simulink model "mcb_open_loop_control_f28379d111"  (R2023b)
settings: Solver=FixedStepDiscrete  StartTime=0.0  StopTime=5  RelTol=1e-3  EnableMultiTasking=on
InitFcn:
  | mcb_open_loop_control_data;
  | target = mcb_SetProcessorDetails('F28379D',PWM_frequency);
  | 
  | %Read inverter logic from 'Configuration' panel on model
  | inverter.EnableLogic = eval(get_param([bdroot '/Open Loop Control/Parameters/Inverter'],'Value'));
values from neighbouring files (symbols this model uses):
  PWM_frequency = eval(get_param([bdroot '/Open Loop Control/Parameters/PWM Frequency'], 'Value'))    [mcb_open_loop_control_data.m]
  Ts = T_pwm    [mcb_open_loop_control_data.m]
undefined symbols (not defined in the file or in its folder): DiscIntNeverNeededParam, Down, GPTRIP1SEL, GPTRIP2SEL, motor, TZ1, TZ2, Up
libraries: c2802xlib x5, simulink x3, mcbcontrolslib x3, svdschedulerlib x2, c280xlib x2, c2837xDlib x1
settings Model: ExtModeTrigDuration=8  Creator=The MathWorks, Inc.  LastModifiedBy=kapis
settings SolverCC: AlgebraicLoopSolver=TrustRegion  AutoInsertRateTranBlk=on
settings DataIOCC: SaveOutput=off  SaveTime=off  ReturnWorkspaceOutputs=off
settings OptimizationCC: DefaultUnderspecifiedDataType=single  EnhancedBackFolding=on  PassReuseOutputArgsAs=Individual arguments  ZeroExternalMemoryAtStartup=off  MaxStackSize=1024  OptimizeBlockOrder=speed  DifferentSizesBufferReuse=on  OptimizationCustomize=off  DenormalBehavior=FlushToZero  EfficientTunableParamExpr=on
settings DebuggingCC: MultiTaskDSMMsg=none  ParameterPrecisionLossMsg=none  ParameterTunabilityLossMsg=error  UnconnectedInputMsg=warning  UnconnectedOutputMsg=warning  UnconnectedLineMsg=warning
settings HardwareCC: ProdBitPerChar=16  ProdBitPerInt=16  ProdBitPerPointer=32  ProdBitPerSizeT=32  ProdBitPerPtrDiffT=32  ProdLargestAtomicInteger=Integer  ProdLargestAtomicFloat=None  ProdWordSize=16  ProdLongLongMode=on  ProdHWDeviceType=Texas Instruments->C2000
settings ModelReferenceCC: EnableRefExpFcnMdlSchedulingChecks=on
settings SFSimCC: MATLABDynamicMemAlloc=off
settings RTWCC: Description=Embedded Coder  SystemTargetFile=ert.tlc  HardwareBoard=TI Delfino F28379D LaunchPad  TemplateMakefile=ert_default_tmf  GenerateReport=on  Toolchain=Texas Instruments Code Composer Studio (C2000)  IncludeHyperlinkInReport=on  GenerateTraceInfo=on  GenerateTraceReport=on  GenerateTraceReportSl=on  GenerateTraceReportSf=on  GenerateTraceReportEml=on  DLArmComputeVersion=19.05
settings CodeAppCC: ForceParamTrailComments=on  IgnoreCustomStorageClasses=off  OperatorAnnotations=on  SimulinkDataObjDesc=on  SFDataObjDesc=on  InsertBlockDesc=on
settings ERTTargetCC: CodeReplacementLibrary=TI C28x  ExtModeStaticAllocSize=10000

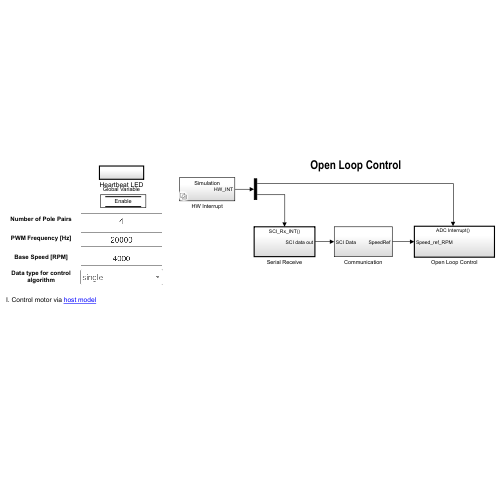
[thumbnail: Simulink's stored preview of the top-level diagram]
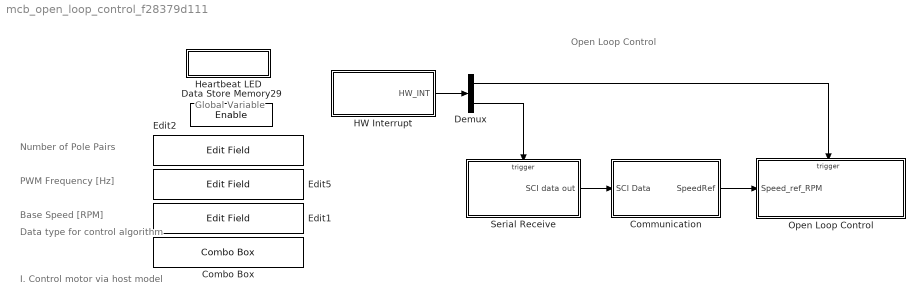
== system mcb_open_loop_control_f28379d111 ==
  note: Open Loop Control
  note: PWM Frequency [Hz]
  note: Base Speed [RPM]
  note: Number of Pole Pairs
  note: Data type for control algorithm
  note: Global Variable
  note: I. Control motor via host model
  Combo Box : ComboBox  LabelPosition=Hide  SelectedLabel=single
      settings: Values={{'single', 'fixdt(1,32,17)'}, [0 1]}
  Communication : Subsystem
  Data Store Memory29 : DataStoreMemory  DataStoreName=Enable  ShowAdditionalParam=off  OutDataTypeStr=boolean
  Demux : Demux  Outputs=2
  Edit1 : EditField  LabelPosition=Hide  ShowInitialText=on  Alignment=Center
  Edit2 : EditField  LabelPosition=Hide  ShowInitialText=on  Alignment=Center
  Edit5 : EditField  LabelPosition=Hide  ShowInitialText=on  Alignment=Center
  HW Interrupt : Subsystem  Variant=on  VariantControlMode=sim codegen switching
  Heartbeat LED : Subsystem  TreatAsAtomicUnit=on
  Open Loop Control : Subsystem
  Serial Receive : Subsystem  SystemSampleTime=1e-3
  wires:
  Demux/2 -> Serial Receive/Trigger
  Demux/1 -> Open Loop Control/Trigger
  Communication/1(SpeedRef) -> Open Loop Control/1(Speed_ref_RPM)
  Serial Receive/1(SCI data out) -> Communication/1(SCI Data)
  HW Interrupt/1(HW_INT) -> Demux/1

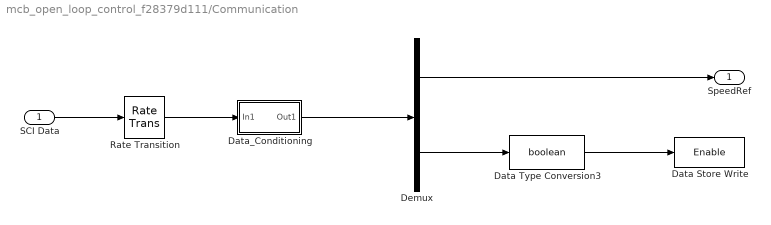
== system mcb_open_loop_control_f28379d111/Communication ==
  SCI Data : Inport
  Data Store Write : DataStoreWrite  DataStoreName=Enable  IndexOptions=Index vector (dialog)  Indices=1  OutputSizes=1
  Data Type Conversion3 : DataTypeConversion  OutDataTypeStr=boolean  RndMeth=Simplest  SaturateOnIntegerOverflow=off
  Data_Conditioning : Subsystem
  Demux : Demux  Outputs=2
  Rate Transition : RateTransition  Deterministic=off  InitialCondition=[1228 0]  OutPortSampleTime=Ts
  SpeedRef : Outport  VectorParamsAs1DForOutWhenUnconnected=off
  wires:
  Rate Transition/1 -> Data_Conditioning/1(In1)
  SCI Data/1 -> Rate Transition/1
  Data_Conditioning/1(Out1) -> Demux/1
  Demux/2 -> Data Type Conversion3/1
  Demux/1 -> SpeedRef/1
  Data Type Conversion3/1 -> Data Store Write/1

== system mcb_open_loop_control_f28379d111/HW Interrupt ==
  Code generation : Subsystem  VariantControl=(codegen)
  Simulation : Subsystem  VariantControl=(sim)
  HW_INT : Outport  OutputFunctionCall=on

== system mcb_open_loop_control_f28379d111/Heartbeat LED ==
  Heartbeat LED : Subsystem  Variant=on  VariantControlMode=sim codegen switching
  RED_LED : Constant  OutDataTypeStr=uint16  SampleTime=0.5
  wires:
  RED_LED/1 -> Heartbeat LED/1(In1)

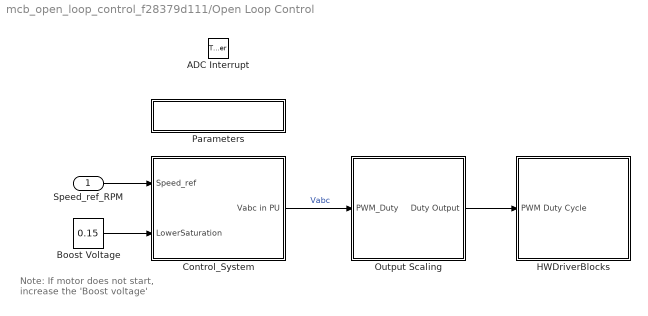
== system mcb_open_loop_control_f28379d111/Open Loop Control ==
  note: Note: If motor does not start, increase the 'Boost voltage'
  Speed_ref_RPM : Inport
  ADC Interrupt : TriggerPort  TriggerType=function-call  VariantControl=Variant
  Boost Voltage : Constant  Value=0.15  OutDataTypeStr=dataType
  Control_System : Subsystem
  HWDriverBlocks : Subsystem  Variant=on  VariantControlMode=sim codegen switching
  Output Scaling : Subsystem
  Parameters : Subsystem
  wires:
  Speed_ref_RPM/1 -> Control_System/1(Speed_ref)
  Control_System/1(Vabc in PU) -> Output Scaling/1(PWM_Duty)  "Vabc"
  Output Scaling/1(Duty Output) -> HWDriverBlocks/1(PWM Duty Cycle)
  Boost Voltage/1 -> Control_System/2(LowerSaturation)

== system mcb_open_loop_control_f28379d111/Serial Receive ==
  SCI_Rx_INT : TriggerPort  TriggerType=function-call  VariantControl=Variant
  SCI_Rx : Subsystem  Variant=on  VariantControlMode=sim codegen switching
  SCI data out : Outport  VectorParamsAs1DForOutWhenUnconnected=off
  wires:
  SCI_Rx/1(Output) -> SCI data out/1

== system mcb_open_loop_control_f28379d111/Communication/Data_Conditioning ==
  In1 : Inport
  Data Type Conversion2 : DataTypeConversion  OutDataTypeStr=int16  ConvertRealWorld=Stored Integer (SI)  RndMeth=Simplest  SaturateOnIntegerOverflow=off
  Out1 : Outport  VectorParamsAs1DForOutWhenUnconnected=off
  wires:
  Data Type Conversion2/1 -> Out1/1
  In1/1 -> Data Type Conversion2/1

== system mcb_open_loop_control_f28379d111/HW Interrupt/Code generation ==
  HWI_ADCB1_INT : svdschedulerlib/Hardware Interrupt v2  ISRGroup=ADC - Analog to Digital Converter  ISRName=ADCA1_INT  ISRNumber=32  NumEventsToServe=1  EventsList={'on','EOC event','1';'off','Overflow event','2';'off','Custom event','3'}  SelectedEvents={'event1'}  TaskPriority=30  DisablePreemption=off  ClearInterruptFlagsAtEndOfEvent=on  InterruptDefinitionFile=$(TARGET_ROOT)/registry/interrupts/F2837xS_interrupts.xml  HardwareBoard=F2837x  EnableSimPort=off
      settings: LibrarySourceBlock=c2000lib/Scheduling/Hardware Interrupt
  HWI_SCIA_RX_INT : svdschedulerlib/Hardware Interrupt v2  ISRGroup=ADC - Analog to Digital Converter  ISRName=ADCA1_INT  ISRNumber=32  NumEventsToServe=1  EventsList={'on','EOC event','1';'off','Overflow event','2';'off','Custom event','3'}  SelectedEvents={'event1'}  TaskPriority=50  DisablePreemption=on  ClearInterruptFlagsAtEndOfEvent=on  InterruptDefinitionFile=$(TARGET_ROOT)/registry/interrupts/F2837xS_interrupts.xml  HardwareBoard=F2837x  EnableSimPort=off
      settings: LibrarySourceBlock=c2000lib/Scheduling/Hardware Interrupt
  Mux : Mux  Inputs=2
  HW_INT : Outport
  wires:
  HWI_ADCB1_INT/1 -> Mux/1
  Mux/1 -> HW_INT/1
  HWI_SCIA_RX_INT/1 -> Mux/2

== system mcb_open_loop_control_f28379d111/HW Interrupt/Simulation ==
  ADCINT1 : simulink/Ports & Subsystems/Function-Call Generator  sample_time=Ts  numberOfIterations=1  DisallowWideOutput=off
  Mux : Mux  Inputs=2
  SCI_Rx_INT : simulink/Ports & Subsystems/Function-Call Generator  sample_time=0.1  numberOfIterations=1  DisallowWideOutput=off
  HW_INT : Outport
  wires:
  SCI_Rx_INT/1 -> Mux/2
  ADCINT1/1 -> Mux/1
  Mux/1 -> HW_INT/1

== system mcb_open_loop_control_f28379d111/Heartbeat LED/Heartbeat LED ==
  In1 : Inport
  Code generation : Subsystem  VariantControl=(codegen)
  Simulation : Subsystem  VariantControl=(sim)

== system mcb_open_loop_control_f28379d111/Open Loop Control/Control_System ==
  Speed_ref : Inport
  LowerSaturation : Inport  Port=2
  SpeedRefToFreq : Subsystem
  VabcCalc : Subsystem
  Vabc in PU : Outport  VectorParamsAs1DForOutWhenUnconnected=off
  wires:
  Speed_ref/1 -> SpeedRefToFreq/1(Speed_Ref)
  SpeedRefToFreq/1(Frequency) -> VabcCalc/1(Frequency)
  VabcCalc/1(Vabc) -> Vabc in PU/1
  LowerSaturation/1 -> VabcCalc/2(LowerSaturation)

== system mcb_open_loop_control_f28379d111/Open Loop Control/HWDriverBlocks ==
  PWM Duty Cycle : Inport
  Codegen : Subsystem  VariantControl=(codegen)
  Sim : Subsystem  VariantControl=(sim)

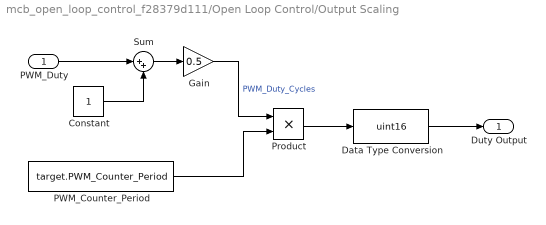
== system mcb_open_loop_control_f28379d111/Open Loop Control/Output Scaling ==
  PWM_Duty : Inport
  Constant : Constant  OutDataTypeStr=dataType
  Data Type Conversion : DataTypeConversion  OutDataTypeStr=uint16  RndMeth=Floor
  Gain : Gain  Gain=0.5  RndMeth=Simplest  OutDataTypeStr=Inherit: Same as input
  PWM_Counter_Period : Constant  Value=target.PWM_Counter_Period  OutDataTypeStr=dataType  SampleTime=-1
  Product : Product  RndMeth=Simplest  OutDataTypeStr=Inherit: Same as first input
  Sum : Sum  Inputs=|++
  Duty Output : Outport
  wires:
  Data Type Conversion/1 -> Duty Output/1
  PWM_Counter_Period/1 -> Product/2
  PWM_Duty/1 -> Sum/1
  Product/1 -> Data Type Conversion/1
  Constant/1 -> Sum/2
  Sum/1 -> Gain/1
  Gain/1 -> Product/1  "PWM_Duty_Cycles"

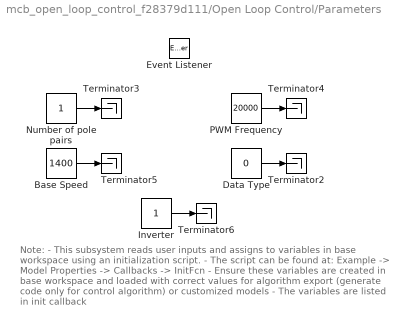
== system mcb_open_loop_control_f28379d111/Open Loop Control/Parameters ==
  note: Note:
      | - This subsystem reads user inputs and assigns to variables
      | in base workspace using an initialization script.
      | - The script can be found at: Example -> Model Properties ->
      | Callbacks -> InitFcn
      | - Ensure these variables are created in base workspace and
      | loaded with correct values for algorithm export (generate
      | code only for control algorithm) or customized models
      | - The variables are listed in init callback
  Base Speed : Constant  Value=1400
  Data Type : Constant  Value=0
  Event Listener : EventListener  DisableCoverage=on  EventName=reset
  Inverter : Constant
  Number of pole pairs : Constant
  PWM Frequency : Constant  Value=20000
  Terminator{2..6} (5 alike) : Terminator
  wires:
  Data Type/1 -> Terminator2/1
  Number of pole pairs/1 -> Terminator3/1
  PWM Frequency/1 -> Terminator4/1
  Base Speed/1 -> Terminator5/1
  Inverter/1 -> Terminator6/1

== system mcb_open_loop_control_f28379d111/Serial Receive/SCI_Rx ==
  Codegen : Subsystem  VariantControl=(codegen)
  Sim : Subsystem  VariantControl=(sim)
  Output : Outport

== system mcb_open_loop_control_f28379d111/Heartbeat LED/Heartbeat LED/Code generation ==
  In1 : Inport
  Digital Output : c2837xDlib/Digital Output  GPIO_Number=GPIO32~GPIO39  GPIO_Bit0=off  GPIO_BIT0_Toggle=on  GPIO_Bit1=off  GPIO_BIT1_Toggle=off  GPIO_Bit2=on  GPIO_BIT2_Toggle=on  GPIO_Bit3=off  GPIO_BIT3_Toggle=off  GPIO_Bit4=off  GPIO_BIT4_Toggle=off  GPIO_Bit5=off  GPIO_BIT5_Toggle=off  GPIO_Bit6=off  GPIO_BIT6_Toggle=off  GPIO_Bit7=off  GPIO_BIT7_Toggle=off
  wires:
  In1/1 -> Digital Output/1

== system mcb_open_loop_control_f28379d111/Heartbeat LED/Heartbeat LED/Simulation ==
  In1 : Inport
  Simulation_Terminator : Terminator
  wires:
  In1/1 -> Simulation_Terminator/1

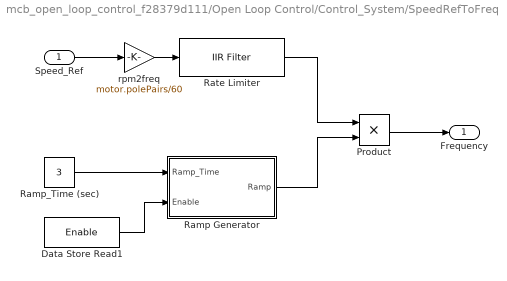
== system mcb_open_loop_control_f28379d111/Open Loop Control/Control_System/SpeedRefToFreq ==
  Speed_Ref : Inport
  Data Store Read1 : DataStoreRead  DataStoreName=Enable  IndexOptions=Index vector (dialog)  Indices=1  OutputSizes=1
  Product : Product  RndMeth=Simplest  OutDataTypeStr=Inherit: Same as first input
  Ramp Generator : Subsystem
  Ramp_Time (sec) : Constant  Value=3  OutDataTypeStr=dataType  SampleTime=-1
  Rate Limiter : mcbcontrolslib/IIR Filter  VariantControl=Low Pass Filter  VariantSelect=Low-pass  Filter_constant=0.0001  advancedSettings=off  Ts=50e-6  cutOff_freq=0.31834
  rpm2freq : Gain  Gain=motor.polePairs/60  OutDataTypeStr=dataType  RndMeth=Simplest
  Frequency : Outport
  wires:
  Product/1 -> Frequency/1
  Ramp Generator/1(Ramp) -> Product/2
  Ramp_Time (sec)/1 -> Ramp Generator/1(Ramp_Time)
  rpm2freq/1 -> Rate Limiter/1
  Data Store Read1/1 -> Ramp Generator/2(Enable)
  Speed_Ref/1 -> rpm2freq/1
  Rate Limiter/1 -> Product/1

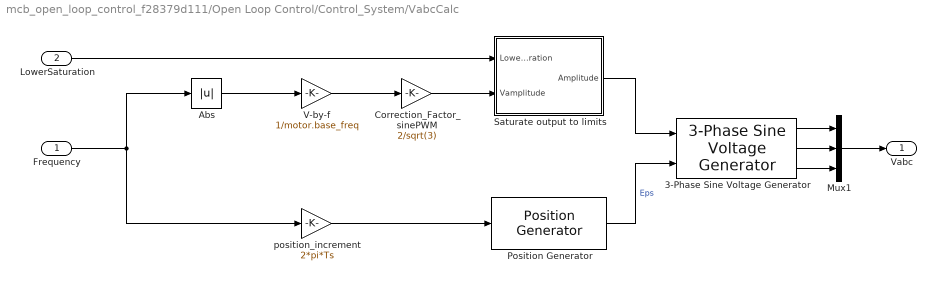
== system mcb_open_loop_control_f28379d111/Open Loop Control/Control_System/VabcCalc ==
  Frequency : Inport
  LowerSaturation : Inport  Port=2
  3-Phase Sine Voltage Generator : mcbcontrolslib/3-Phase Sine Voltage Generator  AngleInput=Radians  N_points=1024
  Abs : Abs  RndMeth=Simplest  SaturateOnIntegerOverflow=off
  Correction_Factor_sinePWM : Gain  Gain=2/sqrt(3)  RndMeth=Simplest  OutDataTypeStr=Inherit: Same as input
  Mux1 : Mux  Inputs=3
  Position Generator : mcbcontrolslib/Position Generator  AngleOutput=Radians  ExternalReset=none  Offset=0
  Saturate output to limits : Subsystem
  V-by-f : Gain  Gain=1/motor.base_freq  RndMeth=Simplest  OutDataTypeStr=Inherit: Same as input
  position_increment : Gain  Gain=2*pi*Ts  RndMeth=Simplest  OutDataTypeStr=Inherit: Same as input
  Vabc : Outport
  wires:
  Frequency/1 -> Abs/1, position_increment/1
  position_increment/1 -> Position Generator/1
  3-Phase Sine Voltage Generator/3 -> Mux1/3
  3-Phase Sine Voltage Generator/2 -> Mux1/2
  V-by-f/1 -> Correction_Factor_sinePWM/1
  3-Phase Sine Voltage Generator/1 -> Mux1/1
  Correction_Factor_sinePWM/1 -> Saturate output to limits/2(Vamplitude)
  Mux1/1 -> Vabc/1
  LowerSaturation/1 -> Saturate output to limits/1(Lower Saturation)
  Saturate output to limits/1(Amplitude) -> 3-Phase Sine Voltage Generator/1
  Position Generator/1 -> 3-Phase Sine Voltage Generator/2  "Eps"
  Abs/1 -> V-by-f/1

== system mcb_open_loop_control_f28379d111/Open Loop Control/HWDriverBlocks/Codegen ==
  PWM Duty Cycle : Inport
  Data Serial Output : Subsystem
  Demux : Demux  Outputs=2
  PWM Output : Subsystem
  Sensors : Subsystem
  wires:
  Demux/1 -> Data Serial Output/1(Data1_Log)
  Sensors/1(Iab_measured_ADC) -> Demux/1
  PWM Duty Cycle/1 -> PWM Output/1(PWM Duty Cycle)
  Demux/2 -> Data Serial Output/2(Data2_Log)

== system mcb_open_loop_control_f28379d111/Open Loop Control/HWDriverBlocks/Sim ==
  PWM Duty Cycle : Inport
  Terminator : Terminator
  wires:
  PWM Duty Cycle/1 -> Terminator/1

== system mcb_open_loop_control_f28379d111/Serial Receive/SCI_Rx/Codegen ==
  SCI Receive : c280xlib/SCI Receive  sciModule=A  dataHead=''  headerCheckMaxCount=16  dataTail=''  dataType=uint16  dataLenOptions=Length via dialog  dataDim=2  maxDataLength=1  initValue=0  errOption=Output the last received value  errValue=0  sampleTime=-1  blockingMode=on  timeOut=0.00875  outputStatus=off
  Output : Outport
  wires:
  SCI Receive/1 -> Output/1

== system mcb_open_loop_control_f28379d111/Serial Receive/SCI_Rx/Sim ==
  Constant : Constant  OutDataTypeStr=dataType
  Data Type Conversion : DataTypeConversion  OutDataTypeStr=int16  RndMeth=Simplest  SaturateOnIntegerOverflow=off
  Data Type Conversion3 : DataTypeConversion  OutDataTypeStr=uint16  ConvertRealWorld=Stored Integer (SI)  RndMeth=Simplest  SaturateOnIntegerOverflow=off
  Mux : Mux  Inputs=2
  Speed_ref_rpm (sim) : Constant  Value=1200  OutDataTypeStr=dataType  SampleTime=-1
  Output : Outport
  wires:
  Mux/1 -> Data Type Conversion/1
  Data Type Conversion3/1 -> Output/1
  Data Type Conversion/1 -> Data Type Conversion3/1
  Constant/1 -> Mux/2
  Speed_ref_rpm (sim)/1 -> Mux/1

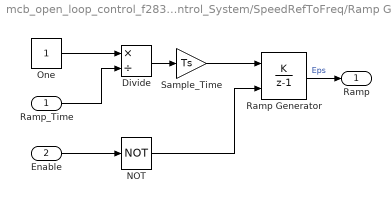
== system mcb_open_loop_control_f28379d111/Open Loop Control/Control_System/SpeedRefToFreq/Ramp Generator ==
  Ramp_Time : Inport
  Enable : Inport  Port=2
  Divide : Product  Inputs=*/  RndMeth=Simplest  OutDataTypeStr=Inherit: Same as first input
  NOT : Logic  Operator=NOT  IconShape=distinctive  AllPortsSameDT=off  OutDataTypeStr=boolean
  One : Constant  OutDataTypeStr=dataType  SampleTime=-1
  Ramp Generator : DiscreteIntegrator  IntegratorMethod=Accumulation: Forward Euler  gainval=1  ExternalReset=sampled level  SampleTime=-1  OutDataTypeStr=dataType  RndMeth=Simplest  LimitOutput=on  UpperSaturationLimit=1  LowerSaturationLimit=0  ICPrevOutput=DiscIntNeverNeededParam  ICPrevScaledInput=DiscIntNeverNeededParam
  Sample_Time : Gain  Gain=Ts  RndMeth=Simplest  OutDataTypeStr=Inherit: Same as input
  Ramp : Outport
  wires:
  Divide/1 -> Sample_Time/1
  Ramp Generator/1 -> Ramp/1  "Eps"
  Sample_Time/1 -> Ramp Generator/1
  One/1 -> Divide/1
  Ramp_Time/1 -> Divide/2
  Enable/1 -> NOT/1
  NOT/1 -> Ramp Generator/2

== system mcb_open_loop_control_f28379d111/Open Loop Control/Control_System/VabcCalc/Saturate output to limits ==
  Lower Saturation : Inport
  Vamplitude : Inport  Port=2
  Relational Operator : RelationalOperator  Operator=>  OutDataTypeStr=boolean  RndMeth=Simplest  InputSameDT=off
  Saturation : Saturate  UpperLimit=0.95  LowerLimit=0  RndMeth=Simplest
  Switch : Switch  Criteria=u2 > Threshold  SaturateOnIntegerOverflow=off  InputSameDT=off
  Amplitude : Outport
  wires:
  Saturation/1 -> Amplitude/1
  Switch/1 -> Saturation/1
  Relational Operator/1 -> Switch/2
  Lower Saturation/1 -> Switch/3, Relational Operator/2
  Vamplitude/1 -> Switch/1, Relational Operator/1

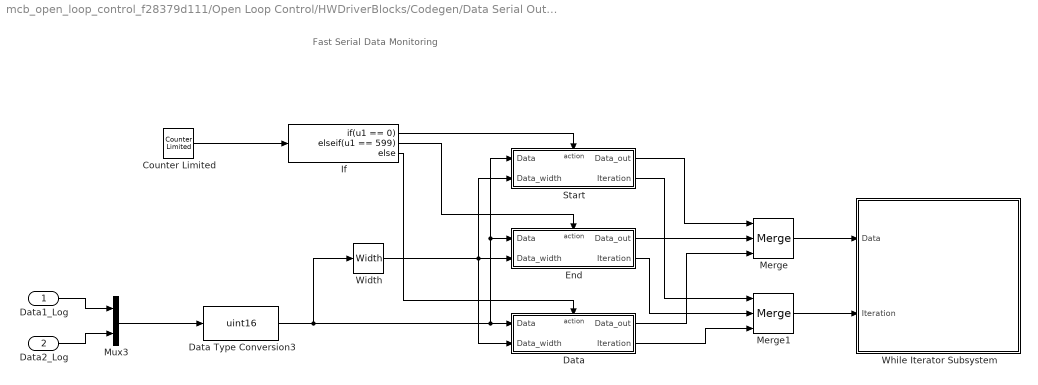
== system mcb_open_loop_control_f28379d111/Open Loop Control/HWDriverBlocks/Codegen/Data Serial Output ==
  note: Fast Serial Data Monitoring
  Data1_Log : Inport
  Data2_Log : Inport  Port=2
  Counter Limited : simulink/Sources/Counter Limited  uplimit=599  tsamp=-1
  Data : Subsystem  TreatAsAtomicUnit=on
  Data Type Conversion3 : DataTypeConversion  OutDataTypeStr=uint16  ConvertRealWorld=Stored Integer (SI)  SaturateOnIntegerOverflow=off  RndMeth=Floor
  End : Subsystem  TreatAsAtomicUnit=on
  If : If  IfExpression=u1 == 0  ElseIfExpressions=u1 == 599
  Merge : Merge  Inputs=3
  Merge1 : Merge  Inputs=3
  Mux3 : Mux  Inputs=2
  Start : Subsystem  TreatAsAtomicUnit=on
  While Iterator Subsystem : Subsystem  TreatAsAtomicUnit=on
  Width : Width  OutDataTypeMode=All ports same datatype  DataType=uint16
  wires:
  Merge/1 -> While Iterator Subsystem/1(Data)
  If/2 -> End/Action
  If/3 -> Data/Action
  Counter Limited/1 -> If/1
  End/1(Data_out) -> Merge/2
  Width/1 -> Data/2(Data_width), Start/2(Data_width), End/2(Data_width)
  Start/1(Data_out) -> Merge/1
  Start/2(Iteration) -> Merge1/1
  Merge1/1 -> While Iterator Subsystem/2(Iteration)
  Data/1(Data_out) -> Merge/3
  If/1 -> Start/Action
  End/2(Iteration) -> Merge1/2
  Data/2(Iteration) -> Merge1/3
  Data Type Conversion3/1 -> Width/1, Start/1(Data), End/1(Data), Data/1(Data)
  Data2_Log/1 -> Mux3/2
  Data1_Log/1 -> Mux3/1
  Mux3/1 -> Data Type Conversion3/1

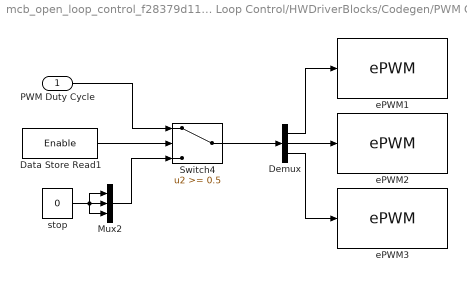
== system mcb_open_loop_control_f28379d111/Open Loop Control/HWDriverBlocks/Codegen/PWM Output ==
  PWM Duty Cycle : Inport
  Data Store Read1 : DataStoreRead  DataStoreName=Enable  IndexOptions=Index vector (dialog)  Indices=1  OutputSizes=1
  Demux : Demux  Outputs=3
  Mux2 : Mux  Inputs=3
  Switch4 : Switch  Threshold=0.5  RndMeth=Simplest  SaturateOnIntegerOverflow=off  InputSameDT=off
  ePWM1 : c2802xlib/ePWM  PwmType=C2000_Type4  useModule=ePWM1  ePWMxLINKTBPRD=Not Linked  periodUnits=Clock cycles  timerSource=Specify via dialog  timerPeriod_clk=target.PWM_Counter_Period  timerPeriod_sec=0.0001  tbshadow=Counter equals to zero  countingMode=Up-Down  phaseActiveEnable=Disable  phaseDirection=Count down after sync  phaseActive=0  synchronizationEnable=off  dcaevt1Sync=off  dcbevt1Sync=off  synchronizationOption=Counter equals to zero (CTR=Zero)  dcbevt1SyncOut=off  dcaevt1SyncOut=off  cmpdSyncOut=off  cmpcSyncOut=off  cmpbSyncOut=off  zeroSyncOut=on  swfSyncOut=off  perSynchronizationOption=Counter equals to period (CTR=PRD)  clockPrescale=1  HSclockPrescale=1  enswap=off  ePWMxAStatus=on  ePWMxAactionLogic1=Do nothing  ePWMxAactionLogic2=Do nothing  ePWMxAactionLogic3=Clear  ePWMxAactionLogic4=Set  ePWMxAactionLogic5=Do nothing  ePWMxAactionLogic6=Do nothing  ePWMxACSFenable=off  ePWMxACSFvalue=Forcing disable  ePWMxASFreload=Zero  ePWMxBStatus=off  ePWMxBactionLogic1=Set  ePWMxBactionLogic2=Clear  ePWMxBactionLogic3=Do nothing  ePWMxBactionLogic4=Do nothing  ePWMxBactionLogic5=Clear  ePWMxBactionLogic6=Set  ePWMxBCSFenable=off  ePWMxBCSFvalue=Forcing disable  ePWMxBSFreload=Zero  ePWNxBOutWay=off  ePWMxLINKCMPA=Not Linked  CMPAUnits=Clock cycles  CMPASource=Input port  CMPAValue_per=50  CMPAValue_clk=floor(target.PWM_Counter_Period/2+1)  enCMPAshadow=Counter equals to zero (CTR=Zero)  ePWMxLINKCMPB=Not Linked  CMPBUnits=Clock cycles  CMPBSource=Specify via dialog  CMPBValue_per=50  CMPBValue_clk=floor(target.PWM_Counter_Period/2+1)  enCMPBshadow=Counter equals to zero (CTR=Zero)  ePWMxLINKCMPC=Not Linked  CMPCUnits=Clock cycles  CMPCSource=Specify via dialog  CMPCValue_per=50  CMPCValue_clk=32000  enCMPCshadow=Counter equals to zero (CTR=Zero)  ePWMxLINKCMPD=Not Linked  CMPDUnits=Clock cycles  CMPDSource=Specify via dialog  CMPDValue_per=50  CMPDValue_clk=32000  enCMPDshadow=Counter equals to zero (CTR=Zero)  enableDBePWMxA=on  enableDBePWMxB=on  enhalfcycle=off  DBpolarity=Active high complementary (AHC)  DBedgeDelay=Positive  DBSource_ePWMxA=ePWMxA  DBSource_ePWMxB=ePWMxA  DBPeriodUnits=Clock cycles  DBperiodSource=Specify via dialog  REDperiod=250  FEDperiod=250  REDperiod_sec=0  FEDperiod_sec=0  LoadModeDBRED=Immediate without using shadow  LoadModeDBFED=Immediate without using shadow  adcstartModuleA=on  adcrequestEventA=First event  adcstartEventA=Digital Compare Module A Event 1 start of conversion (DCAEVT1.soc)  adcstartEventA_type2=Counter equals to period (CTR=PRD)  adcstartModuleB=off  adcrequestEventB=First event  adcstartEventB=Counter equals to zero (CTR=Zero)  adcstartEventB_type2=Counter equals to zero (CTR=Zero)  intEn=off  intPrd=First event  intSel=Counter equals to zero (CTR=Zero)  intSel_type2=Counter equals to zero (CTR=Zero)  hrpe=off  enHRPWM=off  HRPWM_LoadMode=Counter equals to period (CTR=PRD)  HRPWM_CTLMode=Duty or Period control mode  HRPWM_EDGMode=Both edge  hrpeb=off  enHRPWMB=off  HRPWM_LoadModeB=Counter equals to zero (CTR=ZERO)  HRPWM_CTLModeB=Duty or Period control mode  HRPWM_EDGModeB=Both edge  enHRDBRED=off  enHRDBFED=off  enSFO=on  enautoconv=on  chopperEnable=off  chopperFrequency=1  chopperFirstwidth=1  chopperDuty=12.5%  tripZonesource=Specify via dialog  tzselOSHT1=off  tzselOSHT2=off  tzselOSHT3=off  tzselOSHDCAEV1=off  tzselOSHDCBEV1=off  tzselCBC1=off  tzselCBC2=off  tzselCBC3=off  tzselCBCDCAEV2=off  tzselCBCDCBEV2=off  tzselOSHT4=off  tzselOSHT5=off  tzselOSHT6=off  tzselCBC4=off  tzselCBC5=off  tzselCBC6=off  enTzOstIntr=off  enTzCbcIntr=off  enTzDCAEVT1Intr=off  enTzDCAEVT2Intr=off  enTzDCBEVT1Intr=off  enTzDCBEVT2Intr=off  ePWMxAforced=No action  ePWMxBforced=No action  DCAEVT1forced=No action  DCBEVT1forced=No action  DCAEVT2forced=No action  DCBEVT2forced=No action  dcah=Trip Zone 1 input (TZ1)  dcal=Trip Zone 2 input (TZ2)  dcbh=Trip Zone 1 input (TZ1)  dcbl=Trip Zone 2 input (TZ2)  dcah_type2=GPTRIP1SEL/(TZ1)  dcal_type2=GPTRIP2SEL/(TZ2)  dcbh_type2=GPTRIP1SEL/(TZ1)  dcbl_type2=GPTRIP2SEL/(TZ2)  gendcaevt1=Event disabled  gendcaevt2=Event disabled  gendcbevt1=Event disabled  gendcbevt2=Event disabled  dcaevt1src=DCAEVT1 with sync  dcaevt2src=DCAEVT2 with sync  dcbevt1src=DCBEVT1 with sync  dcbevt2src=DCBEVT2 with sync  pulsesel=Counter equals to zero (CTR=Zero)  blankinv=off  blankoffset=0  blankwidth=0  evsrcsel=Filtered version of DCAEVT1 (DCAEVT1FILT)  encape=off
  ePWM2 : c2802xlib/ePWM  PwmType=C2000_Type4  useModule=ePWM2  ePWMxLINKTBPRD=Not Linked  periodUnits=Clock cycles  timerSource=Specify via dialog  timerPeriod_clk=target.PWM_Counter_Period  timerPeriod_sec=0.0001  tbshadow=Counter equals to zero  countingMode=Up-Down  phaseActiveEnable=Set counter to phase value specified via dialog  phaseDirection=Count up after sync  phaseActive=0  synchronizationEnable=off  dcaevt1Sync=off  dcbevt1Sync=off  synchronizationOption=Pass through (EPWMxSYNCI or SWFSYNC)  dcbevt1SyncOut=off  dcaevt1SyncOut=off  cmpdSyncOut=off  cmpcSyncOut=off  cmpbSyncOut=off  zeroSyncOut=off  swfSyncOut=on  perSynchronizationOption=Counter equals to period (CTR=PRD)  clockPrescale=1  HSclockPrescale=1  enswap=off  ePWMxAStatus=on  ePWMxAactionLogic1=Do nothing  ePWMxAactionLogic2=Do nothing  ePWMxAactionLogic3=Clear  ePWMxAactionLogic4=Set  ePWMxAactionLogic5=Do nothing  ePWMxAactionLogic6=Do nothing  ePWMxACSFenable=off  ePWMxACSFvalue=Forcing disable  ePWMxASFreload=Zero  ePWMxBStatus=off  ePWMxBactionLogic1=Set  ePWMxBactionLogic2=Clear  ePWMxBactionLogic3=Do nothing  ePWMxBactionLogic4=Do nothing  ePWMxBactionLogic5=Clear  ePWMxBactionLogic6=Set  ePWMxBCSFenable=off  ePWMxBCSFvalue=Forcing disable  ePWMxBSFreload=Zero  ePWNxBOutWay=off  ePWMxLINKCMPA=Not Linked  CMPAUnits=Clock cycles  CMPASource=Input port  CMPAValue_per=50  CMPAValue_clk=floor(target.PWM_Counter_Period/2+1)  enCMPAshadow=Counter equals to zero (CTR=Zero)  ePWMxLINKCMPB=Not Linked  CMPBUnits=Clock cycles  CMPBSource=Specify via dialog  CMPBValue_per=50  CMPBValue_clk=floor(target.PWM_Counter_Period/2+1)  enCMPBshadow=Counter equals to zero (CTR=Zero)  ePWMxLINKCMPC=Not Linked  CMPCUnits=Clock cycles  CMPCSource=Specify via dialog  CMPCValue_per=50  CMPCValue_clk=32000  enCMPCshadow=Counter equals to zero (CTR=Zero)  ePWMxLINKCMPD=Not Linked  CMPDUnits=Clock cycles  CMPDSource=Specify via dialog  CMPDValue_per=50  CMPDValue_clk=32000  enCMPDshadow=Counter equals to zero (CTR=Zero)  enableDBePWMxA=on  enableDBePWMxB=on  enhalfcycle=off  DBpolarity=Active high complementary (AHC)  DBedgeDelay=Positive  DBSource_ePWMxA=ePWMxA  DBSource_ePWMxB=ePWMxA  DBPeriodUnits=Clock cycles  DBperiodSource=Specify via dialog  REDperiod=250  FEDperiod=250  REDperiod_sec=0  FEDperiod_sec=0  LoadModeDBRED=Immediate without using shadow  LoadModeDBFED=Immediate without using shadow  adcstartModuleA=off  adcrequestEventA=First event  adcstartEventA=Digital Compare Module A Event 1 start of conversion (DCAEVT1.soc)  adcstartEventA_type2=Counter equals to period (CTR=PRD)  adcstartModuleB=off  adcrequestEventB=First event  adcstartEventB=Counter equals to zero (CTR=Zero)  adcstartEventB_type2=Counter equals to zero (CTR=Zero)  intEn=off  intPrd=First event  intSel=Counter equals to zero (CTR=Zero)  intSel_type2=Counter equals to zero (CTR=Zero)  hrpe=off  enHRPWM=off  HRPWM_LoadMode=Counter equals to period (CTR=PRD)  HRPWM_CTLMode=Duty or Period control mode  HRPWM_EDGMode=Both edge  hrpeb=off  enHRPWMB=off  HRPWM_LoadModeB=Counter equals to zero (CTR=ZERO)  HRPWM_CTLModeB=Duty or Period control mode  HRPWM_EDGModeB=Both edge  enHRDBRED=off  enHRDBFED=off  enSFO=on  enautoconv=on  chopperEnable=off  chopperFrequency=1  chopperFirstwidth=1  chopperDuty=12.5%  tripZonesource=Specify via dialog  tzselOSHT1=off  tzselOSHT2=off  tzselOSHT3=off  tzselOSHDCAEV1=off  tzselOSHDCBEV1=off  tzselCBC1=off  tzselCBC2=off  tzselCBC3=off  tzselCBCDCAEV2=off  tzselCBCDCBEV2=off  tzselOSHT4=off  tzselOSHT5=off  tzselOSHT6=off  tzselCBC4=off  tzselCBC5=off  tzselCBC6=off  enTzOstIntr=off  enTzCbcIntr=off  enTzDCAEVT1Intr=off  enTzDCAEVT2Intr=off  enTzDCBEVT1Intr=off  enTzDCBEVT2Intr=off  ePWMxAforced=No action  ePWMxBforced=No action  DCAEVT1forced=No action  DCBEVT1forced=No action  DCAEVT2forced=No action  DCBEVT2forced=No action  dcah=Trip Zone 1 input (TZ1)  dcal=Trip Zone 2 input (TZ2)  dcbh=Trip Zone 1 input (TZ1)  dcbl=Trip Zone 2 input (TZ2)  dcah_type2=GPTRIP1SEL/(TZ1)  dcal_type2=GPTRIP2SEL/(TZ2)  dcbh_type2=GPTRIP1SEL/(TZ1)  dcbl_type2=GPTRIP2SEL/(TZ2)  gendcaevt1=Event disabled  gendcaevt2=Event disabled  gendcbevt1=Event disabled  gendcbevt2=Event disabled  dcaevt1src=DCAEVT1 with sync  dcaevt2src=DCAEVT2 with sync  dcbevt1src=DCBEVT1 with sync  dcbevt2src=DCBEVT2 with sync  pulsesel=Counter equals to zero (CTR=Zero)  blankinv=off  blankoffset=0  blankwidth=0  evsrcsel=Filtered version of DCAEVT1 (DCAEVT1FILT)  encape=off
  ePWM3 : c2802xlib/ePWM  PwmType=C2000_Type4  useModule=ePWM3  ePWMxLINKTBPRD=Not Linked  periodUnits=Clock cycles  timerSource=Specify via dialog  timerPeriod_clk=target.PWM_Counter_Period  timerPeriod_sec=0.0001  tbshadow=Counter equals to zero  countingMode=Up-Down  phaseActiveEnable=Set counter to phase value specified via dialog  phaseDirection=Count up after sync  phaseActive=0  synchronizationEnable=off  dcaevt1Sync=off  dcbevt1Sync=off  synchronizationOption=Pass through (EPWMxSYNCI or SWFSYNC)  dcbevt1SyncOut=off  dcaevt1SyncOut=off  cmpdSyncOut=off  cmpcSyncOut=off  cmpbSyncOut=off  zeroSyncOut=off  swfSyncOut=on  perSynchronizationOption=Counter equals to period (CTR=PRD)  clockPrescale=1  HSclockPrescale=1  enswap=off  ePWMxAStatus=on  ePWMxAactionLogic1=Do nothing  ePWMxAactionLogic2=Do nothing  ePWMxAactionLogic3=Clear  ePWMxAactionLogic4=Set  ePWMxAactionLogic5=Do nothing  ePWMxAactionLogic6=Do nothing  ePWMxACSFenable=off  ePWMxACSFvalue=Forcing disable  ePWMxASFreload=Zero  ePWMxBStatus=off  ePWMxBactionLogic1=Set  ePWMxBactionLogic2=Clear  ePWMxBactionLogic3=Do nothing  ePWMxBactionLogic4=Do nothing  ePWMxBactionLogic5=Clear  ePWMxBactionLogic6=Set  ePWMxBCSFenable=off  ePWMxBCSFvalue=Forcing disable  ePWMxBSFreload=Zero  ePWNxBOutWay=off  ePWMxLINKCMPA=Not Linked  CMPAUnits=Clock cycles  CMPASource=Input port  CMPAValue_per=50  CMPAValue_clk=floor(target.PWM_Counter_Period/2+1)  enCMPAshadow=Counter equals to zero (CTR=Zero)  ePWMxLINKCMPB=Not Linked  CMPBUnits=Clock cycles  CMPBSource=Specify via dialog  CMPBValue_per=50  CMPBValue_clk=floor(target.PWM_Counter_Period/2+1)  enCMPBshadow=Counter equals to zero (CTR=Zero)  ePWMxLINKCMPC=Not Linked  CMPCUnits=Clock cycles  CMPCSource=Specify via dialog  CMPCValue_per=50  CMPCValue_clk=32000  enCMPCshadow=Counter equals to zero (CTR=Zero)  ePWMxLINKCMPD=Not Linked  CMPDUnits=Clock cycles  CMPDSource=Specify via dialog  CMPDValue_per=50  CMPDValue_clk=32000  enCMPDshadow=Counter equals to zero (CTR=Zero)  enableDBePWMxA=on  enableDBePWMxB=on  enhalfcycle=off  DBpolarity=Active high complementary (AHC)  DBedgeDelay=Positive  DBSource_ePWMxA=ePWMxA  DBSource_ePWMxB=ePWMxA  DBPeriodUnits=Clock cycles  DBperiodSource=Specify via dialog  REDperiod=250  FEDperiod=250  REDperiod_sec=0  FEDperiod_sec=0  LoadModeDBRED=Immediate without using shadow  LoadModeDBFED=Immediate without using shadow  adcstartModuleA=off  adcrequestEventA=First event  adcstartEventA=Digital Compare Module A Event 1 start of conversion (DCAEVT1.soc)  adcstartEventA_type2=Counter equals to period (CTR=PRD)  adcstartModuleB=off  adcrequestEventB=First event  adcstartEventB=Counter equals to zero (CTR=Zero)  adcstartEventB_type2=Counter equals to zero (CTR=Zero)  intEn=off  intPrd=First event  intSel=Counter equals to zero (CTR=Zero)  intSel_type2=Counter equals to zero (CTR=Zero)  hrpe=off  enHRPWM=off  HRPWM_LoadMode=Counter equals to period (CTR=PRD)  HRPWM_CTLMode=Duty or Period control mode  HRPWM_EDGMode=Both edge  hrpeb=off  enHRPWMB=off  HRPWM_LoadModeB=Counter equals to zero (CTR=ZERO)  HRPWM_CTLModeB=Duty or Period control mode  HRPWM_EDGModeB=Both edge  enHRDBRED=off  enHRDBFED=off  enSFO=on  enautoconv=on  chopperEnable=off  chopperFrequency=1  chopperFirstwidth=1  chopperDuty=12.5%  tripZonesource=Specify via dialog  tzselOSHT1=off  tzselOSHT2=off  tzselOSHT3=off  tzselOSHDCAEV1=off  tzselOSHDCBEV1=off  tzselCBC1=off  tzselCBC2=off  tzselCBC3=off  tzselCBCDCAEV2=off  tzselCBCDCBEV2=off  tzselOSHT4=off  tzselOSHT5=off  tzselOSHT6=off  tzselCBC4=off  tzselCBC5=off  tzselCBC6=off  enTzOstIntr=off  enTzCbcIntr=off  enTzDCAEVT1Intr=off  enTzDCAEVT2Intr=off  enTzDCBEVT1Intr=off  enTzDCBEVT2Intr=off  ePWMxAforced=No action  ePWMxBforced=No action  DCAEVT1forced=No action  DCBEVT1forced=No action  DCAEVT2forced=No action  DCBEVT2forced=No action  dcah=Trip Zone 1 input (TZ1)  dcal=Trip Zone 2 input (TZ2)  dcbh=Trip Zone 1 input (TZ1)  dcbl=Trip Zone 2 input (TZ2)  dcah_type2=GPTRIP1SEL/(TZ1)  dcal_type2=GPTRIP2SEL/(TZ2)  dcbh_type2=GPTRIP1SEL/(TZ1)  dcbl_type2=GPTRIP2SEL/(TZ2)  gendcaevt1=Event disabled  gendcaevt2=Event disabled  gendcbevt1=Event disabled  gendcbevt2=Event disabled  dcaevt1src=DCAEVT1 with sync  dcaevt2src=DCAEVT2 with sync  dcbevt1src=DCBEVT1 with sync  dcbevt2src=DCBEVT2 with sync  pulsesel=Counter equals to zero (CTR=Zero)  blankinv=off  blankoffset=0  blankwidth=0  evsrcsel=Filtered version of DCAEVT1 (DCAEVT1FILT)  encape=off
  stop : Constant  Value=0  OutDataTypeStr=single
  wires:
  Demux/3 -> ePWM3/1
  Demux/2 -> ePWM2/1
  PWM Duty Cycle/1 -> Switch4/1
  Demux/1 -> ePWM1/1
  stop/1 -> Mux2/3, Mux2/2, Mux2/1
  Switch4/1 -> Demux/1
  Mux2/1 -> Switch4/3
  Data Store Read1/1 -> Switch4/2

== system mcb_open_loop_control_f28379d111/Open Loop Control/HWDriverBlocks/Codegen/Sensors ==
  ADC_B_IN2 : c2802xlib/ADC  blkParamProc=C2000_Type4  ADCModule=A  samplingMode=Single sample mode  ADCResolution=12-bit (Single-ended input)  useSOC1=SOC0  useSOC2=SOC0_SOC1  SOCAcquisitionWindow=15  SOCTriggerSource=ePWM1_ADCSOCA  SOCInterruptTrigger=No ADCINT  Ts=-1  dType=uint16  postInterrupt=on  interruptSel=ADCINT1  ADCINTContinuous=on  endma=off  chdma=1  conv1=ADCINA0  conv2=ADCINA0 and ADCINB0  conv1_Type4=ADCIN3  conv2_Type4=ADCIN0 and ADCIN1
  ADC_C_IN2 : c2802xlib/ADC  blkParamProc=C2000_Type4  ADCModule=C  samplingMode=Single sample mode  ADCResolution=12-bit (Single-ended input)  useSOC1=SOC0  useSOC2=SOC0_SOC1  SOCAcquisitionWindow=15  SOCTriggerSource=ePWM1_ADCSOCA  SOCInterruptTrigger=No ADCINT  Ts=-1  dType=uint16  postInterrupt=off  interruptSel=ADCINT1  ADCINTContinuous=on  endma=off  chdma=1  conv1=ADCINA0  conv2=ADCINA0 and ADCINB0  conv1_Type4=ADCIN2  conv2_Type4=ADCIN0 and ADCIN1
  Data Type Conversion : DataTypeConversion  OutDataTypeStr=int32  ConvertRealWorld=Stored Integer (SI)  SaturateOnIntegerOverflow=off  RndMeth=Floor
  Mux : Mux  Inputs=2
  Iab_measured_ADC : Outport  InitialOutput=0  VectorParamsAs1DForOutWhenUnconnected=off
  wires:
  ADC_C_IN2/1 -> Mux/1
  ADC_B_IN2/1 -> Mux/2
  Mux/1 -> Data Type Conversion/1
  Data Type Conversion/1 -> Iab_measured_ADC/1

== system mcb_open_loop_control_f28379d111/Open Loop Control/HWDriverBlocks/Codegen/Data Serial Output/Data ==
  Data : Inport
  Data_width : Inport  Port=2
  Action Port : ActionPort  ActionPortLabel=else
  Mux : Mux  Inputs=2
  Start : Constant  Value=hex2dec('0000')  OutDataTypeStr=uint16
  Data_out : Outport  VectorParamsAs1DForOutWhenUnconnected=off
  Iteration : Outport  Port=2  VectorParamsAs1DForOutWhenUnconnected=off
  wires:
  Start/1 -> Mux/2
  Mux/1 -> Data_out/1
  Data/1 -> Mux/1
  Data_width/1 -> Iteration/1

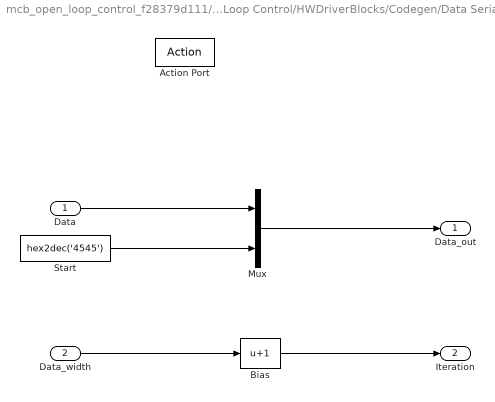
== system mcb_open_loop_control_f28379d111/Open Loop Control/HWDriverBlocks/Codegen/Data Serial Output/End ==
  Data : Inport
  Data_width : Inport  Port=2
  Action Port : ActionPort  ActionPortLabel=elseif(u1 == 599)
  Bias : Bias  Bias=1  SaturateOnIntegerOverflow=off
  Mux : Mux  Inputs=2
  Start : Constant  Value=hex2dec('4545')  OutDataTypeStr=uint16
  Data_out : Outport  VectorParamsAs1DForOutWhenUnconnected=off
  Iteration : Outport  Port=2  VectorParamsAs1DForOutWhenUnconnected=off
  wires:
  Mux/1 -> Data_out/1
  Data_width/1 -> Bias/1
  Start/1 -> Mux/2
  Bias/1 -> Iteration/1
  Data/1 -> Mux/1

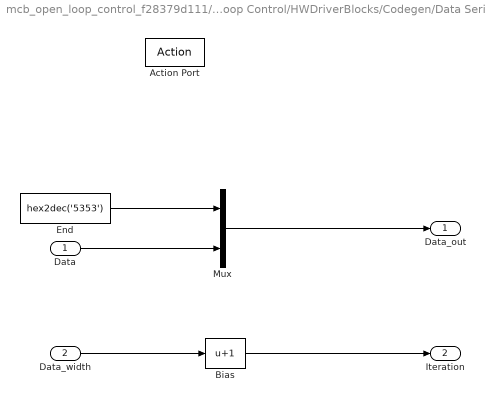
== system mcb_open_loop_control_f28379d111/Open Loop Control/HWDriverBlocks/Codegen/Data Serial Output/Start ==
  Data : Inport
  Data_width : Inport  Port=2
  Action Port : ActionPort  ActionPortLabel=if(u1 == 0)
  Bias : Bias  Bias=1  SaturateOnIntegerOverflow=off
  End : Constant  Value=hex2dec('5353')  OutDataTypeStr=uint16
  Mux : Mux  Inputs=2
  Data_out : Outport  VectorParamsAs1DForOutWhenUnconnected=off
  Iteration : Outport  Port=2  VectorParamsAs1DForOutWhenUnconnected=off
  wires:
  End/1 -> Mux/1
  Mux/1 -> Data_out/1
  Data_width/1 -> Bias/1
  Bias/1 -> Iteration/1
  Data/1 -> Mux/2

== system mcb_open_loop_control_f28379d111/Open Loop Control/HWDriverBlocks/Codegen/Data Serial Output/While Iterator Subsystem ==
  Data : Inport
  Iteration : Inport  Port=2
  Add : Sum  Inputs=+-  OutDataTypeStr=Inherit: Same as first input
  Index Vector : MultiPortSwitch  Inputs=1  SaturateOnIntegerOverflow=off  InputSameDT=off
  SCI Transmit : c280xlib/SCI Transmit  sciModule=A  dataHead=''  dataTail=''  frameSize=1  blockingMode=on  outputStatus=off
  While Iterator : WhileIterator  MaxIters=-1  WhileBlockType=do-while  ShowIterationPort=on  OutputDataType=int16
  wires:
  Iteration/1 -> Add/1
  Add/1 -> While Iterator/1
  Index Vector/1 -> SCI Transmit/1
  Data/1 -> Index Vector/2
  While Iterator/1 -> Index Vector/1, Add/2
